simulink library "vxlib1"  (Simulink 7.6)
settings: Solver=ode45  SolverMode=SingleTasking  StartTime=0.0  StopTime=10.0  RelTol=1e-3
settings Model: Creator=The MathWorks Inc.  ExtModeAutoUpdateStatusClock=off

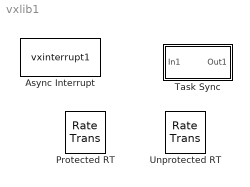
== system vxlib1 ==
  Async Interrupt : S-Function  FunctionName=vxinterrupt1  Parameters=irqnumbers, irqoffsets, irqpriorities, irqpreempts, showinput,manageowntimer,tickres,ticklen  EnableBusSupport=off  mask(VxWorks Interrupt Block){irqnumbers=[1 2], irqoffsets=[192 193], irqpriorities=[10 11], irqpreempts=[0 1], manageowntimer=on, tickres=1/60, ticklen=32bits, showinput=on}
      mask prompts: irqnumbers "VME interrupt number(s):"; irqoffsets "VME interrupt vector offset(s):"; irqpriorities "Simulink task priority(s):"; irqpreempts "Preemption flag(s): preemptable-1, non-preemptable-0"; manageowntimer "Manage own timer"; tickres "Timer resolution (seconds):"; ticklen "Timer size"; showinput "Enable simulation input:"
      mask help: Create VME based Interrupt Service Routine which will execute the downstream subsystem or Task Block.
      mask init:
      | devicedir = fullfile(matlabroot,'rtw','c','tornado','devices');
      | if isempty(findstr(devicedir, path))
      | 	addpath(devicedir);
      | end
      | 
      | irqstr = num2str(irqnumbers);
      | if length(irqstr) ~= 1
      | 	irqstr = 'N';
      | end
      | 
      | if ~showinput
      | 	% make the input port label disappear
      | 	pvalue = irqstr;
      | 	pname = 'output';
      | else
      | 	pvalue = 'SimIRQ';
      | 	pname = 'input';
      | end
      | if strcmp(get_param(bdroot(gcbh),'BlockDiagramType'),'model')
      |   cs = getActiveConfigSet(bdroot);
      |   if isValidParam(cs, 'SampleTimeConstraint') && ...
      | 		  strcmp(get_param(cs, 'SampleTimeConstraint'), 'Specified')
      |     stprop = get_param(cs, 'SampleTimeProperty');
      |     basepriority = stprop(1).Priority;
      |   else
      |     % Simulink default is 40
      |     basepriority = 40;
      |   end
      |   intpris = get_param(gcb,'MaskValues');
      |   pri = eval(intpris{3});
      |   for i=1:length(pri)
      |     if pri(i)>= basepriority
      |       errTxt = ['Interrupt Block ''', gcb, ''' specifies a priority of ''',num2str(pri(i)), ...
      |                 ''' which is lower priority (higher value) or the same as the periodic ', ...
      |                 'base rate priority of ''',num2str(basepriority), '''. Please specify ',...
      |                 'a smaller ''Effective priority'' value.'];
      |       errordlg(errTxt,'Interrupt Priority Error','modal');
      |     end
      |   end
      | end
      mask Help: eval('feval(''rtwprivate'',''rtwhelpview'',''rtw_async_interrupt_block'')');
      mask StyleString: edit,edit,edit,edit,checkbox,edit,popup(32bits|16bits|8bits|auto),checkbox
      mask CallbackString: ||||vxtimercb(gcb);|||
      mask Display:
      | port_label('output',1,['IRQ' irqstr])
      | port_label(pname,1,pvalue)
  Protected RT : RateTransition  Deterministic=off
  Task Sync : Subsystem  mask(VxWorks Task Block){taskname=Task0, taskpriority=50, taskstacksize=8192, parentmanaget=off, tickres=1/60, ticklen=32bits}
      mask prompts: taskname "Task name (10 characters or less):"; taskpriority "Simulink task priority (0-255):"; taskstacksize "Stack size (bytes):"; parentmanaget "Synchronize the data transfer of this task with the caller task"; tickres "Timer resolution (seconds)"; ticklen "Timer size"
      mask help: Creates a Task function which is spawned as a separate VxWorks Task. The Task function runs the code of the downstream function-call subsystem. When this block is run, a semaphore is used to enable the task execution.
      mask init:
      | devicedir = fullfile(matlabroot,'rtw','c','tornado','devices');
      | if isempty(findstr(devicedir, path))
      | 	addpath(devicedir);
      | end
      | 
      | if ~iscvar(taskname)
      |    errordlg('invalid Task Name, first character must be a letter or underscore and remaining characters must be letters,underscores or numbers.','Task Block Error','replace');
      |    taskname = '';
      | end
      mask Help: eval('feval(''rtwprivate'',''rtwhelpview'',''rtw_task_sync_block'')');
      mask StyleString: edit,edit,edit,checkbox,edit,popup(32bits |16bits |8bits |auto)
      mask CallbackString: |||vxtimercb(gcb);||
      mask Display: disp(['Task\n''',taskname,''''])
  Unprotected RT : RateTransition  Integrity=off

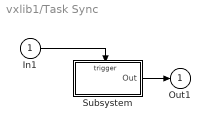
== system vxlib1/Task Sync ==
  In1 : Inport
  Subsystem : Subsystem  TreatAsAtomicUnit=on
      settings: RTWSystemCode=Inline
      mask Type: VxWorks Task Block
  Out1 : Outport
  wires:
  Subsystem/1(Out) -> Out1/1
  In1/1 -> Subsystem/Trigger

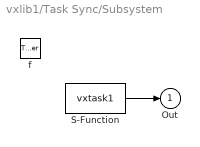
== system vxlib1/Task Sync/Subsystem ==
  f : TriggerPort  TriggerType=function-call
  S-Function : S-Function  FunctionName=vxtask1  Parameters=taskname, taskpriority, taskstacksize, parentmanaget, tickres, ticklen  EnableBusSupport=off
  Out : Outport
  wires:
  S-Function/1 -> Out/1
